simulink model "MotorWithElasticLoads"  (R2015b)
settings: Solver=VariableStepAuto  StartTime=0.0  StopTime=10.0  RelTol=1e-3
values from neighbouring files (symbols this model uses):
  D = 0.01    [MotorWithElasticLoadsConstants.m]
  J = 1    [MotorWithElasticLoadsConstants.m]
  K = 0.5    [MotorWithElasticLoadsConstants.m]
undefined symbols (not defined in the file or in its folder): Jm
settings Model: Creator=kjetil  LastModifiedBy=kjetil

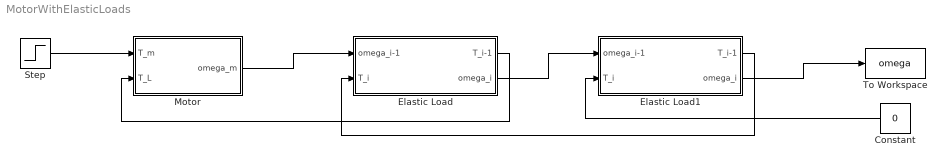
== system MotorWithElasticLoads ==
  Constant : Constant  Value=0
  Elastic Load : Subsystem
  Elastic Load1 : Subsystem
  Motor : Subsystem
  Step : Step  SampleTime=0
  To Workspace : ToWorkspace  VariableName=omega  SaveFormat=Timeseries  SampleTime=-1
  wires:
  Motor/1(omega_m) -> Elastic Load/1(omega_i-1)
  Elastic Load/2(omega_i) -> Elastic Load1/1(omega_i-1)
  Elastic Load/1(T_i-1) -> Motor/2(T_L)
  Elastic Load1/1(T_i-1) -> Elastic Load/2(T_i)
  Constant/1 -> Elastic Load1/2(T_i)
  Step/1 -> Motor/1(T_m)
  Elastic Load1/2(omega_i) -> To Workspace/1

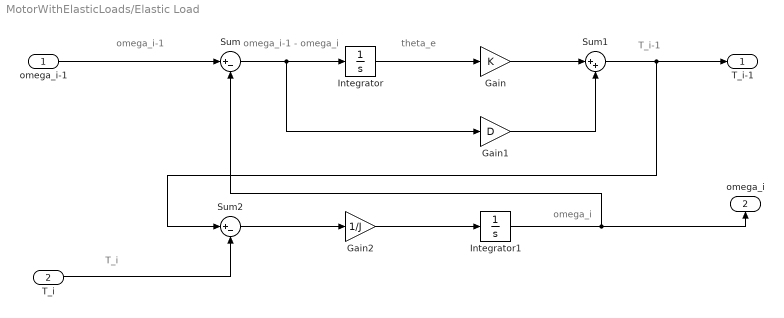
== system MotorWithElasticLoads/Elastic Load ==
  note: omega_i
  note: T_i-1
  note: theta_e
  note: omega_i-1 - omega_i
  note: T_i
  note: omega_i-1
  omega_i-1 : Inport
  T_i : Inport  Port=2
  Gain : Gain  Gain=K
  Gain1 : Gain  Gain=D
  Gain2 : Gain  Gain=1/J
  Integrator : Integrator
  Integrator1 : Integrator
  Sum : Sum  Inputs=|+-
  Sum1 : Sum  Inputs=|++
  Sum2 : Sum  Inputs=|+-
  T_i-1 : Outport
  omega_i : Outport  Port=2
  wires:
  T_i/1 -> Sum2/2
  Sum2/1 -> Gain2/1
  Integrator1/1 -> omega_i/1, Sum/2
  omega_i-1/1 -> Sum/1
  Gain1/1 -> Sum1/2
  Integrator/1 -> Gain/1
  Gain2/1 -> Integrator1/1
  Gain/1 -> Sum1/1
  Sum/1 -> Gain1/1, Integrator/1
  Sum1/1 -> T_i-1/1, Sum2/1

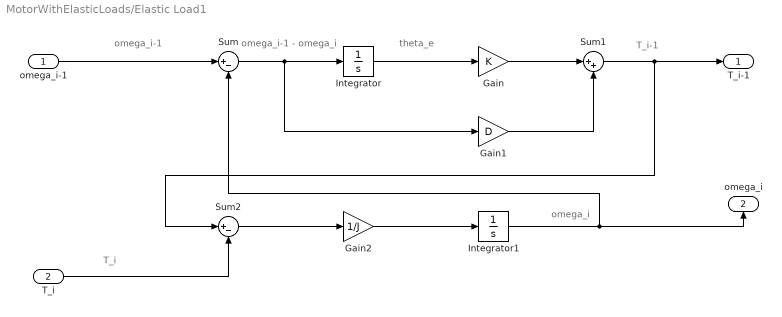
== system MotorWithElasticLoads/Elastic Load1 ==
  note: omega_i
  note: T_i-1
  note: theta_e
  note: omega_i-1 - omega_i
  note: T_i
  note: omega_i-1
  omega_i-1 : Inport
  T_i : Inport  Port=2
  Gain : Gain  Gain=K
  Gain1 : Gain  Gain=D
  Gain2 : Gain  Gain=1/J
  Integrator : Integrator
  Integrator1 : Integrator
  Sum : Sum  Inputs=|+-
  Sum1 : Sum  Inputs=|++
  Sum2 : Sum  Inputs=|+-
  T_i-1 : Outport
  omega_i : Outport  Port=2
  wires:
  T_i/1 -> Sum2/2
  Sum2/1 -> Gain2/1
  Integrator1/1 -> omega_i/1, Sum/2
  omega_i-1/1 -> Sum/1
  Gain1/1 -> Sum1/2
  Integrator/1 -> Gain/1
  Gain2/1 -> Integrator1/1
  Gain/1 -> Sum1/1
  Sum/1 -> Gain1/1, Integrator/1
  Sum1/1 -> T_i-1/1, Sum2/1

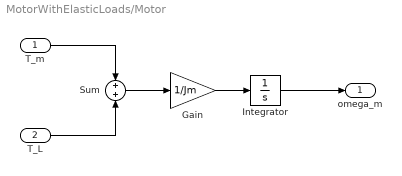
== system MotorWithElasticLoads/Motor ==
  T_m : Inport
  T_L : Inport  Port=2
  Gain : Gain  Gain=1/Jm
  Integrator : Integrator
  Sum : Sum  Inputs=+|+
  omega_m : Outport
  wires:
  Integrator/1 -> omega_m/1
  T_m/1 -> Sum/1
  Sum/1 -> Gain/1
  Gain/1 -> Integrator/1
  T_L/1 -> Sum/2
